simulink model "model"  (Simulink 10.3)
settings: Solver=ode1  StartTime=0.0  StopTime=max(cyc_mph(:,1))  FixedStep=1  MaxStep=1  RelTol=1e-3  AbsTol=1e-3
undefined symbols (not defined in the file): acc_elec_eff, acc_elec_pwr, acc_mech_eff, amb_tmp, cs_charge_deplete_bool, cs_electric_decel_spd, cs_electric_launch_spd_hi, cs_electric_launch_spd_lo, cs_hi_soc, cs_lo_soc, cs_off_trq_frac, cyc_avg_time, cyc_cargo_mass, cyc_elevation_init, cyc_filter_bool, cyc_grade, cyc_mph, ess_module_num, ess_on, ess_voc, ex_calc, ex_cat_co_frac, ex_cat_ext_cp, ex_cat_ext_emisv, ex_cat_ext_init_tmp, ex_cat_ext_mass, ex_cat_ext_sarea, ex_cat_hc_frac, ex_cat_i2p_th_cond, ex_cat_i2x_emisv, ex_cat_i2x_th_cond, ex_cat_int_cp, ex_cat_int_init_tmp, ex_cat_int_mass, ex_cat_int_sarea, ex_cat_lim, ex_cat_m2i_th_cond, ex_cat_m2i_tmp, ex_cat_m2p_emisv, ex_cat_mon_cp, ex_cat_mon_init_tmp, ex_cat_mon_mass, ex_cat_mon_sarea, ex_cat_monf_sarea, ex_cat_moni_sarea, ex_cat_nox_frac, ex_cat_p2x_th_cond, ex_cat_pcm_ecp, ex_cat_pcm_mass, ex_cat_pcm_tmp, ex_cat_pipe_cp, ex_cat_pipe_emisv, ex_cat_pipe_init_tmp, ex_cat_pipe_mass, ex_cat_pipe_sarea, ex_cat_pm_frac, ex_cat_tmp_range, ex_gas_cp, ex_manif_cp, ex_manif_emisv ... (+73)
libraries: lib_controls x6, lib_vehicle x3, lib_accessory x2, lib_interactive x1, lib_energy_storage x1, lib_fuel_converter x1
(part 4 of 5)

== system model/wheel and axle  front/rear <wh>/front/rear brake controller interface (achievable) ==
  F_drivetrain_ach : Inport
  w_wheel_ach : Inport  Port=2
  F_rear_drivetrain_ach : Inport  Port=3
  F_max_front_brake : Inport  Port=4
  F_max_rear_brake : Inport  Port=5
  F_front_brake : Outport  InitialOutput=0
  F_rear_brake : Outport  Port=2  InitialOutput=0
  tag scope: F_drivetrain_ach=global, F_max_front_brake=global, F_max_rear_brake=global, F_rear_drivetrain_ach=global, w_wheel_ach=global
  wires:
  F_rear_drivetrain_ach/1 -> [F_rear_drivetrain_ach]
  F_max_rear_brake/1 -> [F_max_rear_brake]
  F_max_front_brake/1 -> [F_max_front_brake]
  F_drivetrain_ach/1 -> [F_drivetrain_ach]
  w_wheel_ach/1 -> [w_wheel_ach]
  [F_front_brake] -> F_front_brake/1
  [F_rear_brake] -> F_rear_brake/1

== system model/wheel and axle  front/rear <wh>/help ==

== system model/wheel and axle  front/rear <wh>/limits and losses diagnostics ==
  speed : Inport
  front brake : Inport  Port=2
  front brake max : Inport  Port=3
  rear brake max : Inport  Port=4
  rear brake : Inport  Port=5
  Gain : Gain  Gain=-1  SaturateOnIntegerOverflow=on
  Logical Operator : Logic  Operator=OR
  Product : Product  SaturateOnIntegerOverflow=on
  Relational Operator1 : RelationalOperator  Operator===  RndMeth=Nearest  InputSameDT=on
  Relational Operator2 : RelationalOperator  Operator===  RndMeth=Nearest  InputSameDT=on
  Sum3 : Sum  SaturateOnIntegerOverflow=on
  To Workspace6 : ToWorkspace  VariableName=wh_brake_loss_pwr  SampleTime=-1
  tag scope: brake_limited=global
  wires:
  rear brake/1 -> Relational Operator2/2, Sum3/2
  rear brake max/1 -> Relational Operator2/1
  front brake max/1 -> Relational Operator1/2
  front brake/1 -> Relational Operator1/1, Sum3/1
  speed/1 -> Product/1
  Relational Operator2/1 -> Logical Operator/2
  Relational Operator1/1 -> Logical Operator/1
  Logical Operator/1 -> [brake_limited]
  Product/1 -> To Workspace6/1
  Sum3/1 -> Gain/1
  Gain/1 -> Product/2

== system model/wheel and axle  front/rear <wh>/loss (Nm) ==
  note: The loss torque is zero when the axle is not turning.
  axle speed (rad/s) : Inport
  Constant : Constant  Value=0
  Switch : Switch  Threshold=eps  SaturateOnIntegerOverflow=on  InputSameDT=on
  veh mass calc : Subsystem
  wheel & axle bearing drag (Nm) : Lookup  InputValues=wh_axle_loss_mass  Table=wh_axle_loss_trq  SaturateOnIntegerOverflow=on
  drag torque (Nm) : Outport  InitialOutput=0
  wires:
  wheel & axle bearing drag (Nm)/1 -> Switch/1
  Constant/1 -> Switch/3
  axle speed (rad/s)/1 -> Switch/2
  Switch/1 -> drag torque (Nm)/1
  veh mass calc/1(Out1) -> wheel & axle bearing drag (Nm)/1

== system model/wheel and axle  front/rear <wh>/rear brake ==
  F_brake : Inport
  Constant : Constant  Value=wh_max_rear_brake_force
  Terminator : Terminator
  F_brake_max : Outport  InitialOutput=0
  wires:
  F_brake/1 -> Terminator/1
  Constant/1 -> F_brake_max/1

== system model/wheel and axle  front/rear <wh>/rear force ==
  In1 : Inport
  In2 : Inport  Port=2
  Product2 : Product  SaturateOnIntegerOverflow=on
  Sum1 : Sum  Inputs=-+  SaturateOnIntegerOverflow=on
  Sum4 : Sum  Inputs=-+  SaturateOnIntegerOverflow=on
  To Workspace12 : ToWorkspace  VariableName=wh_rear_brake_r  SampleTime=-1
  brake request controller interface1 : Subsystem
  tractive torque req/d of drivetrain (Nm)1 : Gain  Gain=wh_radius  SaturateOnIntegerOverflow=on
  Out1 : Outport
  wires:
  Sum1/1 -> Sum4/2
  Product2/1 -> Sum1/1
  In2/1 -> Product2/2
  In1/1 -> Sum1/2, Product2/1
  tractive torque req/d of drivetrain (Nm)1/1 -> Out1/1
  Sum4/1 -> tractive torque req/d of drivetrain (Nm)1/1
  brake request controller interface1/1(F_rear_brake_req) -> To Workspace12/1, Sum4/1

== system model/wheel and axle  front/rear <wh>/tire slip model (m/s) ==
  note: See note regarding sum in backward path
  weight borne  by front axle (N) : Inport
  total tractive  force available (N) : Inport  Port=2
  axle speed available (rad/s) : Inport  Port=3
  axle speed req'd (rad/s) : Inport  Port=4
  vehicle speed required (m/s) : Inport  Port=5
  weight borne by  rear axle (N) : Inport  Port=6
  front fraction : Inport  Port=7
  Abs1 : Abs  SaturateOnIntegerOverflow=on
  Block NOTES : Subsystem
      mask Display: disp('Block\nNOTES')
  Constant : Constant  Value=1e-3
  Constant5 : Constant
  Constant6 : Constant  Value=wh_radius
  Fcn : Fcn  Expr=1/u
  Relational Operator1 : RelationalOperator  Operator=>  RndMeth=Nearest  InputSameDT=on
  Sum1 : Sum  Inputs=+-  SaturateOnIntegerOverflow=on
  Sum2 : Sum  SaturateOnIntegerOverflow=on
  Sum3 : Sum  SaturateOnIntegerOverflow=on
  Sum4 : Sum  Inputs=-+  SaturateOnIntegerOverflow=on
  Switch1 : Switch  Threshold=eps  SaturateOnIntegerOverflow=on  InputSameDT=on
  front axle : Subsystem
  front frac : Product  SaturateOnIntegerOverflow=on
  rear axle : Subsystem
  vehicle speed (m/s) : Product  Inputs=3  SaturateOnIntegerOverflow=on
  possible vehicle speed (m/s) : Outport  InitialOutput=0
  tag scope: veh_spd_a_rec=global
  wires:
  Sum2/1 -> Sum3/1
  rear axle/1(Out1) -> Sum2/2
  front axle/1(Out1) -> Sum2/1
  Sum1/1 -> rear axle/2(In2)
  front frac/1 -> Sum1/2, front axle/2(In2)
  front fraction/1 -> front frac/2
  total tractive  force available (N)/1 -> Sum1/1, front frac/1
  weight borne by  rear axle (N)/1 -> rear axle/1(In1)
  vehicle speed (m/s)/1 -> [veh_spd_a_rec], Switch1/1
  Switch1/1 -> possible vehicle speed (m/s)/1
  weight borne  by front axle (N)/1 -> front axle/1(In1)
  Abs1/1 -> Relational Operator1/1
  Constant/1 -> Relational Operator1/2
  axle speed req'd (rad/s)/1 -> Sum4/2
  Sum4/1 -> Abs1/1
  vehicle speed required (m/s)/1 -> Switch1/3
  Relational Operator1/1 -> Switch1/2
  Constant6/1 -> vehicle speed (m/s)/3
  axle speed available (rad/s)/1 -> vehicle speed (m/s)/2, Sum4/1
  Constant5/1 -> Sum3/2
  Fcn/1 -> vehicle speed (m/s)/1
  Sum3/1 -> Fcn/1

== system model/wheel and axle  front/rear <wh>/tire slip model (rad/s) ==
  note: Question: for front and rear, is it the sum of or min/max? tm:020703
  note: This block implements the effects of finite tire slip
      | (with respect to the road) on the vehicle speed/wheel speed relationship.
  note: Slip is defined as s=(omega*r - v) / v.  The one-to-one mapping of slip to normalized
      | tractive force, F_tract/W_front_axle, up to the maximum, is stored in the variables
      | "wh_slip" and "wh_slip_force_coeff."
  total tractive  force requested (N) : Inport
  requested time-step average vehicle speed (m/s) : Inport  Port=2
  weight borne by front axle (N) : Inport  Port=3
  weight borne by  rear axle (N)1 : Inport  Port=4
  front traction ratio : Inport  Port=5
  Constant5 : Constant
  Constant6 : Constant  Value=1/wh_radius
  Sum1 : Sum  Inputs=+-  SaturateOnIntegerOverflow=on
  Sum2 : Sum  SaturateOnIntegerOverflow=on
  Sum3 : Sum  SaturateOnIntegerOverflow=on
  To Workspace6 : ToWorkspace  VariableName=wh_slip_r  SampleTime=-1
  front frac : Product  SaturateOnIntegerOverflow=on
  front slip : Subsystem
  rear slip : Subsystem
  wheel speed (rad/s) : Product  Inputs=3  SaturateOnIntegerOverflow=on
  slip-augmented rotational speed (rad/s) : Outport  InitialOutput=0
  wires:
  Sum2/1 -> To Workspace6/1, Sum3/1
  rear slip/1(Out1) -> Sum2/2
  front slip/1(Out1) -> Sum2/1
  weight borne by  rear axle (N)1/1 -> rear slip/1(In1)
  Sum1/1 -> rear slip/2(In2)
  front traction ratio/1 -> front frac/2
  total tractive  force requested (N)/1 -> Sum1/1, front frac/1
  front frac/1 -> front slip/2(In2), Sum1/2
  wheel speed (rad/s)/1 -> slip-augmented rotational speed (rad/s)/1
  Constant5/1 -> Sum3/2
  Sum3/1 -> wheel speed (rad/s)/2
  Constant6/1 -> wheel speed (rad/s)/3
  requested time-step average vehicle speed (m/s)/1 -> wheel speed (rad/s)/1
  weight borne by front axle (N)/1 -> front slip/1(In1)

== system model/wheel and axle  front/rear <wh>/traction controller interface ==
  F_req : Inport
  v_ave_req : Inport  Port=2
  F_req_limited : Outport  InitialOutput=0
  v_req_limited : Outport  Port=2  InitialOutput=0
  wt_front_axle : Outport  Port=3  InitialOutput=0
  wt_rear_axle : Outport  Port=4  InitialOutput=0
  front_traction_ratio : Outport  Port=5  InitialOutput=0
  tag scope: F_req=global, v_ave_req=global
  wires:
  [front_traction_ratio] -> front_traction_ratio/1
  [wt_rear_axle] -> wt_rear_axle/1
  v_ave_req/1 -> [v_ave_req]
  F_req/1 -> [F_req]
  [wt_front_axle] -> wt_front_axle/1
  [v_req_limited] -> v_req_limited/1
  [F_req_limited] -> F_req_limited/1

== system model/<vc> par/engine on (parallel hybrid)/Block NOTES1 ==
  note: This engine state computer keeps the engine on if:
      | [
      | 1) key is on, AND
      | 2) (trq is too high AND speed is too high for idle) OR engine is allowed to idle, AND
      | 3) vehicle speed >= cs_electric_launch_spd [ in m/s ], AND
      | 4) req'd trq > (cs_off_trq_frac * max_trq_at_spd) OR SOC<cs_lo_soc
      | ]
      | OR
      | [ engine was previously on AND the transmission is shifting ]
      |
      | The last condition is added to prevent the engine from unrealistically
      | shutting down for a second or two during a shift.

== system model/<vc> par/engine on (parallel hybrid)/Subsystem ==
  in_1 : Inport
  Clock : Clock
  Constant1 : Constant  Value=n
  Constant2 : Constant
  Integrator : Integrator
  Memory : Memory  InitialCondition=-0.1
  Memory1 : Memory
  Product : Product  Inputs=*/  InputSameDT=on  RndMeth=Zero  SaturateOnIntegerOverflow=on  OutDataTypeStr=Inherit: Same as first input
  Product1 : Product  InputSameDT=on  RndMeth=Zero  SaturateOnIntegerOverflow=on  OutDataTypeStr=Inherit: Same as first input
  Relational Operator : RelationalOperator  Operator=<=  RndMeth=Nearest  InputSameDT=on
  Sum : Sum  Inputs=+-  InputSameDT=on  SaturateOnIntegerOverflow=on  OutDataTypeStr=Inherit: Same as first input
  Sum1 : Sum  Inputs=|+-  InputSameDT=on  SaturateOnIntegerOverflow=on  OutDataTypeStr=Inherit: Same as first input
  Switch{,1..3} (4 alike) : Switch  Threshold=eps  SaturateOnIntegerOverflow=on  InputSameDT=on
  Variable Transport Delay : VariableTransportDelay  MaximumDelay=n
  out_1 : Outport  InitialOutput=0
  wires:
  Product/1 -> out_1/1
  Sum/1 -> Product/1
  Variable Transport Delay/1 -> Sum/2
  Integrator/1 -> Variable Transport Delay/1, Sum/1
  Relational Operator/1 -> Switch/2
  Constant1/1 -> Product1/2
  Clock/1 -> Sum1/1, Memory/1, Relational Operator/1, Switch/1
  Memory/1 -> Sum1/2
  Sum1/1 -> Product1/1
  Product1/1 -> Relational Operator/2, Switch/3
  Switch/1 -> Variable Transport Delay/2, Switch1/2, Switch1/1
  Constant2/1 -> Switch1/3
  Switch1/1 -> Product/2
  Switch2/1 -> Integrator/1
  Switch3/1 -> Memory1/1
  in_1/1 -> Switch2/3, Switch3/3
  Memory1/1 -> Switch2/1, Switch3/1
  [shifting] -> Switch2/2, Switch3/2

== system model/<vc> par/engine on (parallel hybrid)/key_on ==
  Clock : Clock
  Fcn1 : Fcn  Expr=rem(u[1],period)
  Look-Up Table : Lookup  InputValues=t  Table=y  SaturateOnIntegerOverflow=on
  out_1 : Outport  InitialOutput=0
  wires:
  Fcn1/1 -> Look-Up Table/1
  Clock/1 -> Fcn1/1
  Look-Up Table/1 -> out_1/1

== system model/<vc> par/engine on (parallel hybrid)/repeated cycle:  speed required at end of NEXT step ==
  Clock : Clock
  Fcn1 : Fcn  Expr=rem(u[1],period)
  Look-Up Table : Lookup  InputValues=t  Table=y  SaturateOnIntegerOverflow=on
  Memory : Memory  InitialCondition=-0.1
  Sum : Sum  Inputs=+-  InputSameDT=on  SaturateOnIntegerOverflow=on  OutDataTypeStr=Inherit: Same as first input
  Sum1 : Sum  InputSameDT=on  SaturateOnIntegerOverflow=on  OutDataTypeStr=Inherit: Same as first input
  out_1 : Outport  InitialOutput=0
  wires:
  Sum1/1 -> Look-Up Table/1
  Look-Up Table/1 -> out_1/1
  Fcn1/1 -> Sum1/1
  Sum/1 -> Sum1/2
  Memory/1 -> Sum/2
  Clock/1 -> Fcn1/1, Memory/1, Sum/1

== system model/<vc> par/motor controller logic/Block NOTES ==
  note: This block models a motor/controller's logic, modulating the power input requirement as follows:
      | - enforcing the maximum current limit of the motor/controller
      | - shutting the motor off if the average speed over the time step ==0
      | - shutting the motor off if the transmission is shifting.

== system model/<vc> par/motor controller logic/Sign ==
  in_1 : Inport
  Constant : Constant  Value=0
  Relational Operator : RelationalOperator  Operator=>  RndMeth=Nearest  InputSameDT=on
  Relational Operator1 : RelationalOperator  Operator=<  RndMeth=Nearest  InputSameDT=on
  Sum : Sum  Inputs=+-  InputSameDT=on  SaturateOnIntegerOverflow=on  OutDataTypeStr=Inherit: Same as first input
  out_1 : Outport  InitialOutput=0
  wires:
  Sum/1 -> out_1/1
  Relational Operator/1 -> Sum/1
  Relational Operator1/1 -> Sum/2
  Constant/1 -> Relational Operator/2, Relational Operator1/2
  in_1/1 -> Relational Operator1/1, Relational Operator/1

== system model/<vc> par/parallel clutch control/Block NOTES ==
  note: This clutch control block determines the clutch state given the req'd clutch output torque
      | and speed (labelled as gearbox input torque and speed), and the gear number history.
      |                           conditions                                                                       clutch state
      | gear is being shifted OR (trq <~ 0 AND (engine is                                     1 == disengaged
      | clutched to avoid compression braking OR spd < idle))
      |
      | (trq >~ 0) AND (spd < launch speed) AND clutch                                       2 == slipping
      | was not engaged during previous time step
      |
      | neither of above sets of conditions are met                                          3 == engaged
      |
      | But the clutch is always disengaged when the engine is off or was off within the past 0.5 s.

== system model/<vc> par/parallel clutch control/gearbox speed estimator ==
  gb_spd_in_r if no gear change : Inport
  Block NOTES : Subsystem
      mask Display: disp('Block\nNOTES')
  Constant : Constant  Value=eps
  Constant1 : Constant  Value=0
  Constant2 : Constant
  Constant3 : Constant  Value=0.11
  Gain : Gain  Gain=0.447  SaturateOnIntegerOverflow=on  OutDataTypeStr=Inherit: Same as input  ParamDataTypeStr=Inherit: Same as input
  Logical : Logic
  Memory : Memory  InitialCondition=cyc_mph(1,2)*0.447/wh_radius*fd_ratio*gb_ratio(gb_num_init)
  Memory1 : Memory  InitialCondition=1
  Product : Product  Inputs=**/  InputSameDT=on  RndMeth=Zero  SaturateOnIntegerOverflow=on  OutDataTypeStr=Inherit: Same as first input
  Relational : RelationalOperator  Operator=>  RndMeth=Nearest  InputSameDT=on
  Relational1 : RelationalOperator  Operator=<=  RndMeth=Nearest  InputSameDT=on
  Sum : Sum  InputSameDT=on  SaturateOnIntegerOverflow=on  OutDataTypeStr=Inherit: Same as first input
  Sum1 : Sum  Inputs=-+  InputSameDT=on  SaturateOnIntegerOverflow=on  OutDataTypeStr=Inherit: Same as first input
  Switch : Switch  Threshold=eps  SaturateOnIntegerOverflow=on  InputSameDT=on
  Switch1 : Switch  Threshold=eps  SaturateOnIntegerOverflow=on  InputSameDT=on
  dt : Subsystem
  Out1 : Outport
  wires:
  Product/1 -> Switch/1
  Sum/1 -> Product/3
  Gain/1 -> Product/2
  [veh_spd_a_rec] -> Sum/1, Switch/2
  Constant1/1 -> Switch/3
  Memory/1 -> Switch1/1
  Constant/1 -> Sum/2
  [cyc_mph_r] -> Sum1/2
  [mpha] -> Gain/1, Sum1/1
  Constant2/1 -> Relational/2
  Sum1/1 -> Relational/1
  Relational/1 -> Memory1/1
  Switch/1 -> Memory/1
  Switch1/1 -> Out1/1
  gb_spd_in_r if no gear change/1 -> Switch1/3
  [gb_spd_in_a] -> Product/1
  Constant3/1 -> Relational1/2
  Relational1/1 -> Logical/2
  Memory1/1 -> Logical/1
  Logical/1 -> Switch1/2
  dt/1(Out1) -> Relational1/1

== system model/<vc> par/pre-TX parallel gearbox control/Block NOTES ==
  note: This gearbox control block computes the current gear number given the gearbox's
      | req'd output torque and speed and an estimate its efficiency.  Upshifts occur, given a
      | certain engine speed,  when the estimated engine load falls below the upshift curve
      | in engine speed/load space, and downshifts likewise occur when estimated engine
      | load rises above the downshift curve.  Separate upshift and downshift curves are
      | defined for each gear.  An upshift may not be immediately followed by a downshift.
      | If the tires are about to slip, don't upshift unless the engine would be at max. speed.
      | Enforce this rule by setting the load to 1 when the tires are about to slip.

== system model/<vc> par/pre-TX parallel gearbox control/allow downshift? ==
  prev gearnum : Inport
  Logical Operator : Logic  Operator=NOR
  Memory : Memory  InitialCondition=1
  Memory1 : Memory  InitialCondition=1
  Relational Operator1 : RelationalOperator  Operator=>  RndMeth=Nearest  InputSameDT=on
  Relational Operator2 : RelationalOperator  Operator=>  RndMeth=Nearest  InputSameDT=on
  allow shift : Outport  InitialOutput=0
  wires:
  Logical Operator/1 -> allow shift/1
  prev gearnum/1 -> Relational Operator1/1, Memory/1, Relational Operator2/1
  Relational Operator1/1 -> Logical Operator/1
  Memory/1 -> Relational Operator1/2, Memory1/1
  Memory1/1 -> Relational Operator2/2
  Relational Operator2/1 -> Logical Operator/2

== system model/<vc> par/pre-TX parallel gearbox control/allow upshift? ==
  prev gearnum : Inport
  gb_trq_out_r : Inport  Port=2
  gb_spd_out_r : Inport  Port=3
  prev Pout/Pin : Inport  Port=4
  Block NOTES1 : Subsystem
      mask Display: disp('Block\nNOTES')
  Constant : Constant
  Constant1 : Constant  Value=max(mc_map_spd)*mc_spd_scale/tc_mc_to_fc_ratio*.95
  Logical Operator1 : Logic  Operator=OR  Inputs=3
  Memory : Memory  InitialCondition=1
  Product : Product  InputSameDT=on  RndMeth=Zero  SaturateOnIntegerOverflow=on  OutDataTypeStr=Inherit: Same as first input
  Relational Operator : RelationalOperator  Operator=>  RndMeth=Nearest  InputSameDT=on
  Relational Operator1 : RelationalOperator  Operator=>  RndMeth=Nearest  InputSameDT=on
  Saturation : Saturate  UpperLimit=gb_gears_num  LowerLimit=1
  Sum : Sum  InputSameDT=on  SaturateOnIntegerOverflow=on  OutDataTypeStr=Inherit: Same as first input
  est. req'd input pwr (W) : Product  Inputs=**/  InputSameDT=on  RndMeth=Zero  SaturateOnIntegerOverflow=on  OutDataTypeStr=Inherit: Same as first input
  gear ratio : Lookup  InputValues=[1:length(gb_ratio)]  Table=gb_ratio  SaturateOnIntegerOverflow=on
  gear ratio1 : Lookup  InputValues=[1:length(gb_ratio)]  Table=gb_ratio  SaturateOnIntegerOverflow=on
  motor torque capability : Lookup  InputValues=mc_map_spd*mc_spd_scale  Table=mc_max_trq*mc_trq_scale*mc_overtrq_factor+eps  SaturateOnIntegerOverflow=on
  motor (input to gb) pwr capability : Product  InputSameDT=on  RndMeth=Zero  SaturateOnIntegerOverflow=on  OutDataTypeStr=Inherit: Same as first input
  req'd input spd if no gear change : Product  InputSameDT=on  RndMeth=Zero  SaturateOnIntegerOverflow=on  OutDataTypeStr=Inherit: Same as first input
  allow shift : Outport  InitialOutput=0
  wires:
  req'd input spd if no gear change/1 -> Relational Operator1/1
  Constant1/1 -> Relational Operator1/2
  Relational Operator1/1 -> Logical Operator1/3
  gb_spd_out_r/1 -> req'd input spd if no gear change/2, Product/2, est. req'd input pwr (W)/1
  prev gearnum/1 -> gear ratio1/1, Sum/1
  gear ratio1/1 -> req'd input spd if no gear change/1
  Constant/1 -> Sum/2
  Sum/1 -> Saturation/1
  Saturation/1 -> gear ratio/1
  gear ratio/1 -> Product/1
  motor torque capability/1 -> motor (input to gb) pwr capability/2
  Product/1 -> motor torque capability/1, motor (input to gb) pwr capability/1
  motor (input to gb) pwr capability/1 -> Relational Operator/1
  est. req'd input pwr (W)/1 -> Relational Operator/2
  gb_trq_out_r/1 -> est. req'd input pwr (W)/2
  prev Pout/Pin/1 -> est. req'd input pwr (W)/3
  Logical Operator1/1 -> allow shift/1
  Relational Operator/1 -> Logical Operator1/1
  [engine_on] -> Memory/1
  Memory/1 -> Logical Operator1/2

== system model/<vc> par/pre-TX parallel gearbox control/downshift  command ==
  prev gear number : Inport
  engine load : Inport  Port=2
  engine speed : Inport  Port=3
  Mux : Mux  Inputs=2
  Relational Operator : RelationalOperator  Operator=>  RndMeth=Nearest  InputSameDT=on
  load fraction : Subsystem  mask(Gear Selector){spd=gb_dnshift_spd, load=gb_dnshift_load}
      mask prompts: spd "Speeds:"; load "Load Fractions:"
      mask help:
      | This block will perform a linear interplation (extrapolation outside of bounds) to determine the shift point load fraction associated with the current gear number and speed.
      |
      | The Speeds parameter should be defined as an array of vectors containing speeds for each gear number.  The Load Fractions parameter should be defined as a array of vectors containing load fractions indexed by the speeds in the Speeds parameter for each gear number.
      mask Help:
      | Reference the base workspace variables - gb_**shift_spd and gb_**shift_load  where ** is either up for upshift conditions or dn for downshift conditions.
      | 
      | Or define the arrays as follows:
      | 
      | {[spd1 spd2 spd3 spd4]; [spd1 spd2 spd3 spd4]; ...}
      | 
      | {[load1 load2 load3 load4]; [load1 load2 load3 load4]; ...}
      | 
      | where each array contains one row for each gear in the gearbox.  Speeds should be defined in rad/s and loads as a decimal fraction.
  command : Outport  InitialOutput=0
  wires:
  Relational Operator/1 -> command/1
  engine speed/1 -> Mux/2
  prev gear number/1 -> Mux/1
  engine load/1 -> Relational Operator/1
  Mux/1 -> load fraction/1(In1)
  load fraction/1(Out1) -> Relational Operator/2

== system model/<vc> par/pre-TX parallel gearbox control/gearbox speed estimator ==
  gb_spd_in_r if no gear change : Inport
  Block NOTES : Subsystem
      mask Display: disp('Block\nNOTES')
  Constant : Constant  Value=eps
  Constant1 : Constant  Value=0
  Constant2 : Constant  Value=2
  Constant3 : Constant  Value=0.11
  Gain : Gain  Gain=0.447  SaturateOnIntegerOverflow=on  OutDataTypeStr=Inherit: Same as input  ParamDataTypeStr=Inherit: Same as input
  Logical : Logic
  Memory : Memory  InitialCondition=cyc_mph(1,2)*0.447/wh_radius*fd_ratio*gb_ratio(gb_num_init)
  Memory1 : Memory  InitialCondition=1
  Product : Product  Inputs=**/  InputSameDT=on  RndMeth=Zero  SaturateOnIntegerOverflow=on  OutDataTypeStr=Inherit: Same as first input
  Relational : RelationalOperator  Operator=>  RndMeth=Nearest  InputSameDT=on
  Relational1 : RelationalOperator  Operator=<=  RndMeth=Nearest  InputSameDT=on
  Sum : Sum  InputSameDT=on  SaturateOnIntegerOverflow=on  OutDataTypeStr=Inherit: Same as first input
  Sum1 : Sum  Inputs=-+  InputSameDT=on  SaturateOnIntegerOverflow=on  OutDataTypeStr=Inherit: Same as first input
  Switch : Switch  Threshold=eps  SaturateOnIntegerOverflow=on  InputSameDT=on
  Switch1 : Switch  Threshold=eps  SaturateOnIntegerOverflow=on  InputSameDT=on
  dt : Subsystem
  Out1 : Outport
  wires:
  Product/1 -> Switch/1
  Sum/1 -> Product/3
  Gain/1 -> Product/2
  [veh_spd_a_rec] -> Sum/1, Switch/2
  Constant1/1 -> Switch/3
  Memory/1 -> Switch1/1
  Constant/1 -> Sum/2
  [cyc_mph_r] -> Sum1/2
  [mpha] -> Gain/1, Sum1/1
  Constant2/1 -> Relational/2
  Sum1/1 -> Relational/1
  Relational/1 -> Memory1/1
  Switch/1 -> Memory/1
  Switch1/1 -> Out1/1
  gb_spd_in_r if no gear change/1 -> Switch1/3
  [gb_spd_in_a] -> Product/1
  Constant3/1 -> Relational1/2
  Relational1/1 -> Logical/2
  Memory1/1 -> Logical/1
  Logical/1 -> Switch1/2
  dt/1(Out1) -> Relational1/1

== system model/<vc> par/pre-TX parallel gearbox control/shifting1 ==
  gear number : Inport
  Constant : Constant  Value=gb_shift_delay-1e-6
  Relational Operator : RelationalOperator  Operator=<  RndMeth=Nearest  InputSameDT=on
  time since last shift : Subsystem
      mask Display: disp('time since\nlast shift')
  out_1 : Outport  InitialOutput=0
  wires:
  time since last shift/1(out_1) -> Relational Operator/1
  Constant/1 -> Relational Operator/2
  gear number/1 -> time since last shift/1(in_1)
  Relational Operator/1 -> out_1/1

== system model/<vc> par/pre-TX parallel gearbox control/upshift  command ==
  prev gear number : Inport
  engine load : Inport  Port=2
  engine speed : Inport  Port=3
  Mux : Mux  Inputs=2
  Relational Operator : RelationalOperator  Operator=<  RndMeth=Nearest  InputSameDT=on
  load fraction : Subsystem  mask(Gear Selector){spd=gb_upshift_spd, load=gb_upshift_load}
      mask prompts: spd "Speeds:"; load "Load Fractions:"
      mask help:
      | This block will perform a linear interplation (extrapolation outside of bounds) to determine the shift point load fraction associated with the current gear number and speed.
      |
      | The Speeds parameter should be defined as an array of vectors containing speeds for each gear number.  The Load Fractions parameter should be defined as a array of vectors containing load fractions indexed by the speeds in the Speeds parameter for each gear number.
      mask Help:
      | Reference the base workspace variables - gb_**shift_spd and gb_**shift_load  where ** is either up for upshift conditions or dn for downshift conditions.
      | 
      | Or define the arrays as follows:
      | 
      | {[spd1 spd2 spd3 spd4]; [spd1 spd2 spd3 spd4]; ...}
      | 
      | {[load1 load2 load3 load4]; [load1 load2 load3 load4]; ...}
      | 
      | where each array contains one row for each gear in the gearbox.  Speeds should be defined in rad/s and loads as a decimal fraction.
  command : Outport  InitialOutput=0
  wires:
  Relational Operator/1 -> command/1
  engine speed/1 -> Mux/2
  Mux/1 -> load fraction/1(In1)
  prev gear number/1 -> Mux/1
  engine load/1 -> Relational Operator/1
  load fraction/1(Out1) -> Relational Operator/2

== system model/drive cycle <cyc>/distance travelled (m)/Block NOTES ==
  note: This block calculates the distance travelled by the
      |  vehicle based on the achieved speed.

== system model/drive cycle <cyc>/super-smooth, no-lag trace/Subsystem ==
  in_1 : Inport
  Constant1 : Constant  Value=n
  Integrator : Integrator
  Product : Product  Inputs=*/  InputSameDT=on  RndMeth=Zero  SaturateOnIntegerOverflow=on  OutDataTypeStr=Inherit: Same as first input
  Sum : Sum  Inputs=+-  InputSameDT=on  SaturateOnIntegerOverflow=on  OutDataTypeStr=Inherit: Same as first input
  Transport Delay : TransportDelay  DelayTime=n
  out_1 : Outport  InitialOutput=0
  wires:
  Integrator/1 -> Sum/1, Transport Delay/1
  Transport Delay/1 -> Sum/2
  Sum/1 -> Product/1
  in_1/1 -> Integrator/1
  Product/1 -> out_1/1
  Constant1/1 -> Product/2

== system model/drive cycle <cyc>/super-smooth, no-lag trace/repeated cycle ==
  Clock : Clock
  Fcn1 : Fcn  Expr=rem(u+avgtime*0.75,period)
  Look-Up Table : Lookup  InputValues=t  Table=y  SaturateOnIntegerOverflow=on
  out_1 : Outport  InitialOutput=0
  wires:
  Fcn1/1 -> Look-Up Table/1
  Clock/1 -> Fcn1/1
  Look-Up Table/1 -> out_1/1

== system model/electric acc loads <acc>/Electrical Accessory Loads v2 <acc>/Accessory SDO ==
  data bus : Inport
  Demux : Demux  Outputs=3
      settings: DisplayOption=none
  To Workspace : ToWorkspace  VariableName=acc_elec_pwr_r  SampleTime=-1
  To Workspace3 : ToWorkspace  VariableName=acc_elec_pwr_a  SampleTime=-1
  To Workspace4 : ToWorkspace  VariableName=acc_elec_pwr_est  SampleTime=-1
  electrical power logging : Subsystem  mask{eff=acc_mech_eff}
      mask prompts: eff "efficiency of accessory systems (decimal)"
  wires:
  Demux/3 -> To Workspace4/1
  Demux/2 -> electrical power logging/1(In1), To Workspace3/1
  Demux/1 -> To Workspace/1
  data bus/1 -> Demux/1

== system model/electric acc loads <acc>/Electrical Accessory Loads v2 <acc>/Block NOTES ==
  note: This is the electrical auxiliary loads model.
  note: In terms of an interface, the model assumes electrical power generated from
      | a powersource (or powersources)
      |
      | This model takes in requested driveline electrical power output requests and
      | augments power to account for electrically driven accessories.
      |
      | The power passed along down to the driveline is only power to move the
      | vehicle.

== system model/electric acc loads <acc>/Electrical Accessory Loads v2 <acc>/backward model ==
  note: Power Electrical
      | Accessory
      | (W)
  note: P, W, for driveline
  note: Pwr, W, powersource out
  pwr_in : Inport
  on/off : Inport  Port=2
  Constant : Constant  Value=load_on
  Product : Product  Inputs=***  InputSameDT=on  RndMeth=Zero  SaturateOnIntegerOverflow=on  OutDataTypeStr=Inherit: Same as first input
  Sum : Sum  Inputs=|++  InputSameDT=on  SaturateOnIntegerOverflow=on  OutDataTypeStr=Inherit: Same as first input
  electrical accessories (W) : Subsystem  BlockChoice=Electrical Accessories: Time Variable
      settings: AttributesFormatString=%<BlockChoice>  TemplateBlock=lib_accessory/electrical accessories (W)  MemberBlocks=Electrical Accessories: Constant,Electrical Accessories: Time Variable
      mask Display: image(imread('bdi_acc_elec_cs.bmp'))
  elec_out : Outport
  elec_acc_out : Outport  Port=2
  wires:
  Product/1 -> Sum/2, elec_acc_out/1
  Constant/1 -> Product/3
  on/off/1 -> Product/2
  electrical accessories (W)/1(P_elec_acc) -> Product/1
  pwr_in/1 -> Sum/1
  Sum/1 -> elec_out/1

== system model/electric acc loads <acc>/Electrical Accessory Loads v2 <acc>/forward model ==
  note: ASSUMPTIONS
  note: This calculation assumes that the power provider is never so power limited as to
      | not be able to provide at least the value of acc_pwr_in.
  note: electric
      | accessory
      | power (W)
  note: Power Available
  note: Power to driveline
  pwr_in : Inport
  acc_pwr_in : Inport  Port=2
  Sum : Sum  Inputs=|+-  InputSameDT=on  SaturateOnIntegerOverflow=on  OutDataTypeStr=Inherit: Same as first input
  pwr_out : Outport
  acc_pwr_out : Outport  Port=2
  wires:
  acc_pwr_in/1 -> acc_pwr_out/1, Sum/2
  pwr_in/1 -> Sum/1
  Sum/1 -> pwr_out/1

== system model/exhaust sys <ex>/ex gas heat flow/Block NOTES ==
  note: EXHAUST GAS HEAT TRANSFER
      | This block models the heat loss from the exhaust gas as it flows from the engine through the manifold,
      | downpipe, and catalytic converter.  Also included is the increase in gas temperature within the converter
      | due to the catalysis of HC, CO, and NOx. The block is conditionally executed only if engine_on=1.

== system model/exhaust sys <ex>/ex gas heat flow/converter ==
  h,exg : Inport
  Cexg : Inport  Port=2
  Texgi : Inport  Port=3
  Tex : Inport  Port=4
  " Q/C" : Product  Inputs=/*  SaturateOnIntegerOverflow=on
  1/A : Gain  Gain=1/(ex_cat_moni_sarea+ex_cat_int_sarea-ex_cat_mon_sarea)  SaturateOnIntegerOverflow=on
  Demux3 : Demux  Outputs=2
  MinMax : MinMax  Inputs=2
  Mux16 : Mux
  Qci2g_ : Fcn  Expr=u(1)*(ex_cat_int_sarea - ex_cat_mon_sarea)*(u(3)-u(4))
  Qcm2g_ : Fcn  Expr=u(1)*ex_cat_moni_sarea*(u(2)-u(4))
  Selector3 : Selector  InputPortWidth=5  IndexOptions=Index vector (dialog)  Indices=[ 1 2 ]  OutputSizes=1
  T : Sum  SaturateOnIntegerOverflow=on
  T1 : Sum  SaturateOnIntegerOverflow=on
  Texgo : Outport  OutputWhenDisabled=reset  InitialOutput=amb_tmp
  Qcm2g : Outport  Port=2  OutputWhenDisabled=reset  InitialOutput=0
  Qci2g : Outport  Port=3  OutputWhenDisabled=reset  InitialOutput=0
  wires:
  Cexg/1 -> " Q/C"/1, 1/A/1
  h,exg/1 -> MinMax/2
  1/A/1 -> MinMax/1
  MinMax/1 -> Mux16/1
  Tex/1 -> Selector3/1
  Selector3/1 -> Demux3/1
  Demux3/1 -> Mux16/2
  Demux3/2 -> Mux16/3
  Texgi/1 -> T/2, Mux16/4
  Mux16/1 -> Qcm2g_/1, Qci2g_/1
  Qci2g_/1 -> T1/2, Qci2g/1
  Qcm2g_/1 -> T1/1, Qcm2g/1
  " Q/C"/1 -> T/1
  T1/1 -> " Q/C"/2
  T/1 -> Texgo/1

== system model/exhaust sys <ex>/ex gas heat flow/inlet pipe ==
  h,exg : Inport
  Cexg : Inport  Port=2
  Texgi : Inport  Port=3
  Tex : Inport  Port=4
  " Q/C" : Product  Inputs=/*  SaturateOnIntegerOverflow=on
  A : Gain  Gain=ex_cat_pipe_sarea  SaturateOnIntegerOverflow=on
  Memory : Memory  InitialCondition=cyc_mph(1,2)*.447
  MinMax : MinMax  Inputs=2
  Mux19 : Mux  Inputs=3
  Selector2 : Selector  InputPortWidth=5  IndexOptions=Index vector (dialog)  Indices=3  OutputSizes=1
  T : Sum  SaturateOnIntegerOverflow=on
  Ts-Tex,ave : Fcn  Expr=u(2) - (u(3)+u(1))/2
  tailpipe  emis : Product  SaturateOnIntegerOverflow=on
  Texgo : Outport  OutputWhenDisabled=reset  InitialOutput=amb_tmp
  tag scope: Qp2g=global, Tgpo=global
  wires:
  h,exg/1 -> A/1
  MinMax/1 -> tailpipe  emis/1
  A/1 -> MinMax/2
  Cexg/1 -> MinMax/1, " Q/C"/1
  tailpipe  emis/1 -> " Q/C"/2, [Qp2g]
  " Q/C"/1 -> T/1
  Texgi/1 -> T/2, Mux19/1
  T/1 -> Texgo/1, [Tgpo], Memory/1
  Tex/1 -> Selector2/1
  Mux19/1 -> Ts-Tex,ave/1
  Ts-Tex,ave/1 -> tailpipe  emis/2
  Selector2/1 -> Mux19/2
  Memory/1 -> Mux19/3

== system model/exhaust sys <ex>/ex gas heat flow/manifold  ==
  h,exg : Inport
  Cexg : Inport  Port=2
  Texgi : Inport  Port=3
  Tex : Inport  Port=4
  " Q/C" : Product  Inputs=/*  SaturateOnIntegerOverflow=on
  A : Gain  Gain=ex_manif_sarea  SaturateOnIntegerOverflow=on
  Memory : Memory  InitialCondition=cyc_mph(1,2)*.447
  MinMax : MinMax  Inputs=2
  Mux19 : Mux  Inputs=3
  Selector1 : Selector  InputPortWidth=5  IndexOptions=Index vector (dialog)  Indices=5  OutputSizes=1
  T : Sum  SaturateOnIntegerOverflow=on
  Ts-Tex,ave : Fcn  Expr=u(2) - (u(3)+u(1))/2
  tailpipe  emis : Product  SaturateOnIntegerOverflow=on
  Texgo : Outport  OutputWhenDisabled=reset  InitialOutput=amb_tmp
  tag scope: Qma2g=global, Tgmo=global
  wires:
  h,exg/1 -> A/1
  MinMax/1 -> tailpipe  emis/1
  A/1 -> MinMax/2
  Cexg/1 -> MinMax/1, " Q/C"/1
  " Q/C"/1 -> T/1
  T/1 -> [Tgmo], Texgo/1, Memory/1
  tailpipe  emis/1 -> " Q/C"/2, [Qma2g]
  Tex/1 -> Selector1/1
  Selector1/1 -> Mux19/2
  Mux19/1 -> Ts-Tex,ave/1
  Memory/1 -> Mux19/3
  Ts-Tex,ave/1 -> tailpipe  emis/2
  Texgi/1 -> Mux19/1, T/2

== system model/exhaust sys <ex>/ex sys heat flow/Block NOTES ==
  note: CATALYTIC CONVERTER HEAT LOSS
      | This block models the heat loss from a catalytic converter (conventional or vacuum-insulated).
      | Convection (as a function of vehicle speed), radiation, and conduction effects are included.
      | Converter monolith (m), interior (i), pipe (p), and exterior (x) and engine manifold
      | heat flows are estimated based on the temperatures from the previous iteration.

== system model/exhaust sys <ex>/removal efficiencies/removal efficiencies (base ADVISOR) ==
  Ex Cat T (C) : Inport
  Enable : EnablePort  StatesWhenEnabling=reset
  CO temp eff : Lookup  InputValues=ex_cat_tmp_range  Table=ex_cat_co_frac  SaturateOnIntegerOverflow=on
  HC temp eff : Lookup  InputValues=ex_cat_tmp_range  Table=ex_cat_hc_frac  SaturateOnIntegerOverflow=on
  Mux : Mux
  NOx temp eff : Lookup  InputValues=ex_cat_tmp_range  Table=ex_cat_nox_frac  SaturateOnIntegerOverflow=on
  PM temp eff : Lookup  InputValues=ex_cat_tmp_range  Table=ex_cat_pm_frac  SaturateOnIntegerOverflow=on
  removal effs : Outport  OutputWhenDisabled=reset  InitialOutput=0
  wires:
  Ex Cat T (C)/1 -> PM temp eff/1, NOx temp eff/1, CO temp eff/1, HC temp eff/1
  Mux/1 -> removal effs/1
  PM temp eff/1 -> Mux/4
  NOx temp eff/1 -> Mux/3
  HC temp eff/1 -> Mux/1
  CO temp eff/1 -> Mux/2

== system model/exhaust sys <ex>/removal efficiencies/removal efficiencies ORNL ==
  gas_flow (g/s) : Inport
  Ex Gas T (C) : Inport  Port=2
  O2_exh (g/s) : Inport  Port=3
  emis Engine Out (g/s) : Inport  Port=4
  Ex Cat T (C) : Inport  Port=5
  Enable : EnablePort  StatesWhenEnabling=reset
  CO : Terminator
  CO-Conversion : Subsystem
  Constant : Constant  Value=1200
  Demux : Demux
  HC-Conversion : Subsystem
  Mux : Mux
  NOx_Eff : Subsystem
  PM : Terminator
  PM temp eff : Lookup  InputValues=ex_cat_tmp_range  Table=ex_cat_pm_frac  SaturateOnIntegerOverflow=on
  Product : Product  Inputs=/*  SaturateOnIntegerOverflow=on
  Volume  Flow (m^3/sec) : Gain  Gain=2.96E6  SaturateOnIntegerOverflow=on
  removal effs : Outport  OutputWhenDisabled=reset  InitialOutput=0
  wires:
  Mux/1 -> removal effs/1
  gas_flow (g/s)/1 -> CO-Conversion/4(ex_gas_flow), HC-Conversion/4(ex_gas_flow), Product/2
  Ex Cat T (C)/1 -> PM temp eff/1
  O2_exh (g/s)/1 -> CO-Conversion/3(O2_exh), HC-Conversion/3(O2_exh)
  CO-Conversion/1(CO_eff) -> Mux/2
  HC-Conversion/1(HC_eff) -> Mux/1
  NOx_Eff/1(NOx_eff) -> Mux/3
  PM temp eff/1 -> Mux/4
  Ex Gas T (C)/1 -> NOx_Eff/2(Ex_temp), CO-Conversion/2(T_exh), HC-Conversion/2(T_exh)
  Volume  Flow (m^3/sec)/1 -> NOx_Eff/1(vol_flow), CO-Conversion/1(vol_flow), HC-Conversion/1(vol_flow)
  Demux/1 -> NOx_Eff/3(HC_Inlet)
  Demux/3 -> NOx_Eff/4(NOx_Inlet)
  Demux/2 -> CO/1
  Demux/4 -> PM/1
  emis Engine Out (g/s)/1 -> Demux/1
  Constant/1 -> Product/1
  Product/1 -> Volume  Flow (m^3/sec)/1

== system model/fuel converter  <fc>/engine speed estimator/Block NOTES ==
  note: If the clutch is engaged and the trace was missed in the previous time step:
      | The estimated engine speed for the current time step is the actual engine
      | speed from the previous time step.
      |
      | If the clutch is disengaged and the speed is commanded to increase (spin up):
      | The engine speed is the lesser of the commanded speed and the maximum
      | speed attainable given the engine capability.
      |
      | If the clutch is disengaged at the speed is commanded to decrease (spin down):
      | The engine speed is computed by integrating with respect to time the ratio of
      |  closed-throttle torque to engine inertia.
      |
      | Otherwise:
      | The engine speed is equal to the speed command, but no greater than the
      | engine's maximum speed nor less than the engine's idle speed (if the engine is on.)

== system model/fuel converter  <fc>/engine speed estimator/dt ==
  Clock : Clock
  Memory1 : Memory  InitialCondition=-0.1
  Sum1 : Sum  Inputs=+-  InputSameDT=on  SaturateOnIntegerOverflow=on  OutDataTypeStr=Inherit: Same as first input
  out_1 : Outport  InitialOutput=0
  wires:
  Sum1/1 -> out_1/1
  Memory1/1 -> Sum1/2
  Clock/1 -> Memory1/1, Sum1/1

== system model/fuel converter  <fc>/engine speed estimator/effect of inertia (Nm) ==
  req'd spd (rad/s) : Inport
  prev spd : Inport  Port=2
  Clock : Clock
  Constant : Constant  Value=fc_inertia
  Memory : Memory  InitialCondition=-0.1
  Product1 : Product  Inputs=**/  InputSameDT=on  RndMeth=Zero  SaturateOnIntegerOverflow=on  OutDataTypeStr=Inherit: Same as first input
  Sum : Sum  Inputs=+-  InputSameDT=on  SaturateOnIntegerOverflow=on  OutDataTypeStr=Inherit: Same as first input
  Sum1 : Sum  Inputs=+-  InputSameDT=on  SaturateOnIntegerOverflow=on  OutDataTypeStr=Inherit: Same as first input
  (Nm) : Outport  InitialOutput=0
  wires:
  Constant/1 -> Product1/1
  Clock/1 -> Sum1/1, Memory/1
  Memory/1 -> Sum1/2
  Product1/1 -> (Nm)/1
  prev spd/1 -> Sum/2
  req'd spd (rad/s)/1 -> Sum/1
  Sum1/1 -> Product1/3
  Sum/1 -> Product1/2

== system model/fuel converter  <fc>/engine speed estimator/just started spin-down/spin-up ==
  state : Inport
  Logical Operator : Logic
  Logical Operator1 : Logic  Operator=NOT  Inputs=1
  Memory1 : Memory  InitialCondition=1
  trigger : Outport  InitialOutput=0
  wires:
  state/1 -> Memory1/1, Logical Operator/1
  Logical Operator/1 -> trigger/1
  Logical Operator1/1 -> Logical Operator/2
  Memory1/1 -> Logical Operator1/1

== system model/fuel converter  <fc>/engine speed estimator/no-lag Reset Integrator ==
  in_1 : Inport
  in_2 : Inport  Port=2
  in_3 : Inport  Port=3
  Constant : Constant  Value=0
  Memory : Memory  InitialCondition=initval
  Product : Product  InputSameDT=on  RndMeth=Zero  SaturateOnIntegerOverflow=on  OutDataTypeStr=Inherit: Same as first input
  Sum : Sum  InputSameDT=on  SaturateOnIntegerOverflow=on  OutDataTypeStr=Inherit: Same as first input
  Switch : Switch  Threshold=eps  SaturateOnIntegerOverflow=on  InputSameDT=on
  dt : Subsystem
  in_2==0 : RelationalOperator  Operator===  RndMeth=Nearest  InputSameDT=on
  out_1 : Outport  InitialOutput=0
  wires:
  Constant/1 -> in_2==0/2
  in_2==0/1 -> Switch/2
  Switch/1 -> Memory/1, out_1/1
  Sum/1 -> Switch/1
  Memory/1 -> Sum/1
  Product/1 -> Sum/2
  dt/1(out_1) -> Product/1
  in_1/1 -> Product/2
  in_2/1 -> in_2==0/1
  in_3/1 -> Switch/3

== system model/fuel converter  <fc>/engine torque/Block NOTES ==
  note: If the engine is not spinning down with the clutch disengaged:
      | 1.  Engine brake (aka map) torque is given by the required shaft
      | torque plus enough torque to accelerate the engine's rotating
      | parts as commanded and torque to power the accessories,
      | subject to the engine's torque limits at the current speed.
      | 2.  Shaft torque is engine brake torque less the effects of inertia
      | and accessories.
      |
      | If the engine is spinning down:
      | 1.  Engine brake/map torque is the closed-throttle torque.
      | 2.  Shaft torque is zero.

== system model/fuel converter  <fc>/engine torque/T_closed throttle ==
  w_APU : Inport
  Saturation : Saturate  UpperLimit=max(fc_map_spd)*fc_spd_scale  LowerLimit=min(fc_map_spd)*fc_spd_scale
  ctt lookup : Lookup  InputValues=fc_map_spd*fc_spd_scale  Table=fc_ct_trq*fc_trq_scale  SaturateOnIntegerOverflow=on
  T_closed throttle : Outport  InitialOutput=0
  wires:
  w_APU/1 -> Saturation/1
  Saturation/1 -> ctt lookup/1
  ctt lookup/1 -> T_closed throttle/1

== system model/fuel converter  <fc>/engine torque/T_max ==
  w_APU : Inport
  Saturation1 : Saturate  UpperLimit=max(fc_map_spd)*fc_spd_scale  LowerLimit=min(fc_map_spd)*fc_spd_scale
  max_torque lookup : Lookup  InputValues=fc_map_spd*fc_spd_scale  Table=fc_max_trq*fc_trq_scale  SaturateOnIntegerOverflow=on
  T_max : Outport  InitialOutput=0
  tag scope: engine_rpm=global
  wires:
  Saturation1/1 -> [engine_rpm], max_torque lookup/1
  max_torque lookup/1 -> T_max/1
  w_APU/1 -> Saturation1/1

== system model/fuel converter  <fc>/engine torque/effect of inertia (Nm) ==
  engine spd (rad/s) : Inport
  >=0 : Saturate  UpperLimit=inf  LowerLimit=0
  Block NOTES : Subsystem
      mask Display: disp('Block\nNOTES')
  Clock : Clock
  Constant : Constant  Value=fc_inertia
  Constant1 : Constant  Value=max(fc_max_trq)*fc_trq_scale
  Constant2 : Constant  Value=0.01
  Memory : Memory  InitialCondition=-0.1
  Memory1 : Memory  InitialCondition=vc_idle_spd*vc_key_on(1,2)
  Memory2 : Memory
  MinMax : MinMax  Inputs=2  InputSameDT=on  SaturateOnIntegerOverflow=on
  Product : Product  InputSameDT=on  RndMeth=Zero  SaturateOnIntegerOverflow=on  OutDataTypeStr=Inherit: Same as first input
  Product1 : Product  Inputs=*/*  InputSameDT=on  RndMeth=Zero  SaturateOnIntegerOverflow=on  OutDataTypeStr=Inherit: Same as first input
  Relational : RelationalOperator  Operator=>  RndMeth=Nearest  InputSameDT=on
  Sum : Sum  Inputs=+-  InputSameDT=on  SaturateOnIntegerOverflow=on  OutDataTypeStr=Inherit: Same as first input
  Sum1 : Sum  Inputs=+-  InputSameDT=on  SaturateOnIntegerOverflow=on  OutDataTypeStr=Inherit: Same as first input
  Sum2 : Sum  Inputs=-+  InputSameDT=on  SaturateOnIntegerOverflow=on  OutDataTypeStr=Inherit: Same as first input
  Switch : Switch  Threshold=eps  SaturateOnIntegerOverflow=on  InputSameDT=on
  engine inertia as a function of total vehicle inertia (generous approximation) : Subsystem
  (Nm) : Outport  InitialOutput=0
  wires:
  engine spd (rad/s)/1 -> Sum/1, Memory1/1
  Constant2/1 -> Relational/2
  Sum2/1 -> Relational/1
  >=0/1 -> Switch/1
  Relational/1 -> Memory2/1
  Memory2/1 -> Switch/2
  Clock/1 -> Sum1/1, Memory/1
  Memory/1 -> Sum1/2
  Constant/1 -> Product1/3
  Sum1/1 -> Product1/2
  Switch/1 -> Product1/1
  [mpha] -> Sum2/1
  [cyc_mph_r] -> Sum2/2
  MinMax/1 -> (Nm)/1
  Product1/1 -> MinMax/2
  engine inertia as a function of total vehicle inertia (generous approximation)/1(Out1) -> Product/1
  Constant1/1 -> Product/2
  Product/1 -> MinMax/1
  Memory1/1 -> Sum/2
  Sum/1 -> Switch/3, >=0/1

== system model/gearbox <gb>/Pout/Pin, neglecting inertia/Pout/Pin (neglecting inertia) ==
  in_1 : Inport
  in_2 : Inport  Port=2
  Fcn : Fcn  Expr=1/u
  Product : Product  SaturateOnIntegerOverflow=on
  out_1 : Outport  InitialOutput=0
  wires:
  in_1/1 -> Product/1
  Fcn/1 -> Product/2
  Product/1 -> out_1/1
  in_2/1 -> Fcn/1

== system model/gearbox <gb>/Pout/Pin, neglecting inertia/make division bombproof ==
  note: only add eps if Tin-Tinertia is == 0 (this avoids problems when Tin-Tineratia == -eps
      | which happens from time to time
  Tin-Tinertia : Inport
  Block NOTES : Subsystem
      mask Display: disp('Block\nNOTES')
  Constant : Constant  Value=eps
  Constant1 : Constant  Value=0
  Product : Product  SaturateOnIntegerOverflow=on
  Relational Operator1 : RelationalOperator  Operator===  RndMeth=Nearest  InputSameDT=on
  make division bombproof : Sum  SaturateOnIntegerOverflow=on
  Out1 : Outport
  wires:
  Tin-Tinertia/1 -> make division bombproof/1, Relational Operator1/1
  Constant1/1 -> Relational Operator1/2
  Product/1 -> make division bombproof/2
  Relational Operator1/1 -> Product/1
  Constant/1 -> Product/2
  make division bombproof/1 -> Out1/1

== system model/gearbox <gb>/loss (Nm)/3D discrete lookup table (sfun) ==
  lookup speed (rad/s) : Inport
  lookup trq (Nm) : Inport  Port=2
  "gear_number  (e.g., 1, 2, 3)" : Inport  Port=3
  Mux : Mux  Inputs=3
  Saturation : Saturate  UpperLimit=max(tx_map_spd)  LowerLimit=min(tx_map_spd)
  Saturation1 : Saturate  UpperLimit=max(tx_map_trq)  LowerLimit=min(tx_map_trq)
  Saturation2 : Saturate  UpperLimit=size(tx_eff_map,3)  LowerLimit=1
  discrete interp2d : S-Function  FunctionName=sfun_discreteLookup3d  Parameters=tx_map_trq, tx_map_spd, tx_eff_map  SFunctionDeploymentMode=off  EnableBusSupport=off
  tx_eff : Outport
  wires:
  discrete interp2d/1 -> tx_eff/1
  Mux/1 -> discrete interp2d/1
  lookup speed (rad/s)/1 -> Saturation/1
  Saturation/1 -> Mux/1
  lookup trq (Nm)/1 -> Saturation1/1
  Saturation1/1 -> Mux/2
  "gear_number  (e.g., 1, 2, 3)"/1 -> Saturation2/1
  Saturation2/1 -> Mux/3

== system model/gearbox <gb>/loss (Nm)/Block NOTES ==
  note: 09/20/02:tm modifed lower input to switch after T_loss_at_input to pass the
      | total torque input as the loss when tx_eff=0
      | 5 July 2001:mpo changing loss block to a lookup table methodology
      | 12/20/00:tm revised loss saturation block. lower limit changed
      | from 1 to 0 and upper limit changed from 100 to inf to prevent over or under penalties
  note: Revision Notes:

== system model/mechanical accessory loads <acc>/Mechanical Accessory Loads v2 <acc>/Accessory SDO ==
  data bus : Inport
  Demux : Demux  Outputs=6
      settings: DisplayOption=none
  To Workspace : ToWorkspace  VariableName=acc_mech_trq_r  SampleTime=-1
  To Workspace1 : ToWorkspace  VariableName=acc_mech_pwr_a  SampleTime=-1
  To Workspace2 : ToWorkspace  VariableName=acc_mech_trq_est  SampleTime=-1
  To Workspace3 : ToWorkspace  VariableName=acc_mech_pwr_r  SampleTime=-1
  To Workspace4 : ToWorkspace  VariableName=acc_mech_trq_a  SampleTime=-1
  To Workspace5 : ToWorkspace  VariableName=acc_mech_pwr_est  SampleTime=-1
  mechanical power logging : Subsystem  mask{eff=acc_mech_eff}
      mask prompts: eff "efficiency of accessory systems (decimal)"
  wires:
  Demux/6 -> To Workspace5/1
  Demux/5 -> To Workspace2/1
  Demux/3 -> To Workspace4/1
  Demux/2 -> To Workspace3/1
  Demux/1 -> To Workspace/1
  Demux/4 -> To Workspace1/1, mechanical power logging/1(In1)
  data bus/1 -> Demux/1

== system model/mechanical accessory loads <acc>/Mechanical Accessory Loads v2 <acc>/Block NOTES ==
  note: In this model, only one speed is used to predict accessory
      | loading. The forward model is "dummied" out.
  note: A third input is given for accessory load speed. This is done so that
      | the accessory block can use fc_spd_est which is an estimated vehicle speed
      | (equal to fc_spd_out under normal circumstances).
      | Using fc_spd_est provides total compatibility with ADVISOR v3.2
  note: In terms of an interface, the model assumes belt-driven mechanical loads
      | that run off of a prime mover shaft (e.g., engine shaft)
      |
      | This model takes in requested driveline torque and speed requests and
      | augments torque due to belt driven accessories.
      |
      | The torque passed along down to the driveline is only torque to move the
      | vehicle.
  note: This is the mechanical auxiliary loads model.
